simulink model "la_2dof_ctrl_obs"  (R2019b)
settings: Solver=FixedStepAuto  StartTime=0.0  StopTime=inf  FixedStep=0.001  RelTol=1e-3
model workspace (MAT data in the model file):
  SL_ROS_VariableLengthArrays_MaxSizes.CommonInfo.ArrayTruncateAction = 'EmitWarning'
  SL_ROS_VariableLengthArrays_MaxSizes.MsgTypeMap = containers.Map
  SL_ROS_VariableLengthArrays_MaxSizes.MsgTypeMap.serialization.keys = {'std_msgs/Float64MultiArray'}
  SL_ROS_VariableLengthArrays_MaxSizes.MsgTypeMap.serialization.values{1}.PropertyName = 'Data'
  SL_ROS_VariableLengthArrays_MaxSizes.MsgTypeMap.serialization.values{1}.DataType = 'double'
  SL_ROS_VariableLengthArrays_MaxSizes.MsgTypeMap.serialization.values{1}.MaxLength = 2
  SL_ROS_VariableLengthArrays_MaxSizes.MsgTypeMap.serialization.uniformity = 0
  SL_ROS_VariableLengthArrays_MaxSizes.MsgTypeMap.serialization.keyType = 'char'
  SL_ROS_VariableLengthArrays_MaxSizes.MsgTypeMap.serialization.valueType = 'any'
undefined symbols (not defined in the file): Data, Data_SL_Info
libraries: robotlib x6
settings Model: EnablePacing=on  Creator=markthemagnificent  LastModifiedBy=marco
settings OptimizationCC: EnhancedBackFolding=on  PassReuseOutputArgsAs=Individual arguments  ZeroExternalMemoryAtStartup=off  ZeroInternalMemoryAtStartup=off  MaxStackSize=64  OptimizeBlockOrder=speed  DifferentSizesBufferReuse=on  OptimizationCustomize=off  EfficientTunableParamExpr=on
settings DebuggingCC: ParameterTunabilityLossMsg=error
settings HardwareCC: ProdBitPerLong=64  ProdHWDeviceType=Intel->x86-64 (Linux 64)
settings SFSimCC: MATLABDynamicMemAlloc=off
settings RTWCC: SystemTargetFile=ert.tlc  HardwareBoard=Robot Operating System (ROS)  TLCOptions="-aInlineSetEventsForThisBaseRateFcn=TLC_FALSE -aSuppressMultiTaskScheduler=TLC_FALSE  -aRateBasedStepFcn=0"  TemplateMakefile=ert_default_tmf  GenerateReport=on  Toolchain=Catkin  IncludeHyperlinkInReport=on  LaunchReport=on  TargetLang=C++  GenerateTraceInfo=on  GenerateTraceReport=on  GenerateTraceReportSl=on  GenerateTraceReportSf=on  GenerateTraceReportEml=on
settings CodeAppCC: ForceParamTrailComments=on  IgnoreCustomStorageClasses=off  OperatorAnnotations=on  SimulinkDataObjDesc=on  SFDataObjDesc=on  InsertBlockDesc=on
settings ERTTargetCC: SupportContinuousTime=on

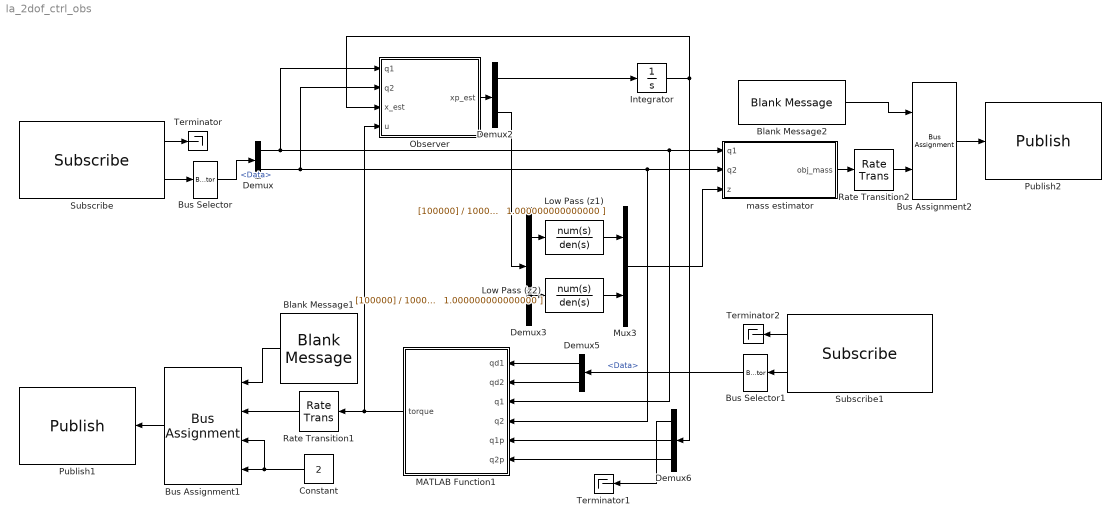
== system la_2dof_ctrl_obs ==
  Blank Message1 : robotlib/Blank Message  messageClass=Message  entityType=std_msgs/Float64MultiArray  messageType=std_msgs/Float64MultiArray  SampleTime=0.001
      settings: SourceProductName=ROS Toolbox
  Blank Message2 : robotlib/Blank Message  messageClass=Message  entityType=std_msgs/Float64  messageType=std_msgs/Float64  SampleTime=0.001
      settings: SourceProductName=ROS Toolbox
  Bus Assignment1 : BusAssignment  AssignedSignals=Data,Data_SL_Info.CurrentLength,Data_SL_Info.ReceivedLength
  Bus Assignment2 : BusAssignment  AssignedSignals=Data
  Bus Selector : BusSelector  OutputSignals=Data
  Bus Selector1 : BusSelector  OutputSignals=Data
  Constant : Constant  Value=2  OutDataTypeStr=uint32  SampleTime=0.001
  Demux : Demux  Outputs=2
  Demux2 : Demux  Outputs=[4,2]
  Demux3 : Demux  Outputs=2
  Demux5 : Demux  Outputs=2
  Demux6 : Demux  Outputs=[2,1,1]
  Integrator : Integrator  InitialCondition=[0 0 0 0]
  Low Pass (z1) : TransferFcn  Numerator=[100000]  Denominator=|
      | 100000*[0.000010000000000   0.000323606797750   0.005236067977500   0.052360679774998   0.323606797749979   1.000000000000000
      | ]
  Low Pass (z2) : TransferFcn  Numerator=[100000]  Denominator=|
      | 100000*[0.000010000000000   0.000323606797750   0.005236067977500   0.052360679774998   0.323606797749979   1.000000000000000
      | ]
  MATLAB Function1 : MATLAB Function  TreatAsAtomicUnit=on
  Mux3 : Mux  Inputs=2
  Observer : MATLAB Function  TreatAsAtomicUnit=on
  Publish1 : robotlib/Publish  topicSource=Specify your own  topic=/hardware/la_torque  messageType=std_msgs/Float64MultiArray  messageQueueLength=1
      settings: SourceProductName=ROS Toolbox
  Publish2 : robotlib/Publish  topicSource=Specify your own  topic=/hardware/la_estimated_mass  messageType=std_msgs/Float64  messageQueueLength=1
      settings: SourceProductName=ROS Toolbox
  Rate Transition1 : RateTransition
  Rate Transition2 : RateTransition
  Subscribe : robotlib/Subscribe  topicSource=Specify your own  topic=/hardware/la_current_pose  messageType=std_msgs/Float64MultiArray  sampleTime=0.001  messageQueueLength=1
      settings: SourceProductName=ROS Toolbox
  Subscribe1 : robotlib/Subscribe  topicSource=Specify your own  topic=/hardware/la_goal_pose  messageType=std_msgs/Float64MultiArray  sampleTime=0.001  messageQueueLength=1
      settings: SourceProductName=ROS Toolbox
  Terminator : Terminator
  Terminator1 : Terminator
  Terminator2 : Terminator
  mass estimator : MATLAB Function  TreatAsAtomicUnit=on
  wires:
  Integrator/1 -> Observer/3(x_est), Demux6/1
  Demux3/1 -> Low Pass (z1)/1
  Demux/2 -> MATLAB Function1/4(q2), mass estimator/2(q2), Observer/2(q2)
  Demux2/2 -> Demux3/1
  Demux2/1 -> Integrator/1
  Observer/1(xp_est) -> Demux2/1
  Demux3/2 -> Low Pass (z2)/1
  Low Pass (z1)/1 -> Mux3/1
  Low Pass (z2)/1 -> Mux3/2
  Mux3/1 -> mass estimator/3(z)
  MATLAB Function1/1(torque) -> Rate Transition1/1, Observer/4(u)
  Demux5/1 -> MATLAB Function1/1(qd1)
  Demux5/2 -> MATLAB Function1/2(qd2)
  Demux/1 -> MATLAB Function1/3(q1), mass estimator/1(q1), Observer/1(q1)
  Demux6/1 -> Terminator1/1
  Demux6/2 -> MATLAB Function1/5(q1p)
  Demux6/3 -> MATLAB Function1/6(q2p)
  Subscribe/1 -> Terminator/1
  Bus Selector/1 -> Demux/1  "<Data>"
  Subscribe/2 -> Bus Selector/1
  Subscribe1/1 -> Terminator2/1
  Subscribe1/2 -> Bus Selector1/1
  Bus Selector1/1 -> Demux5/1  "<Data>"
  Bus Assignment1/1 -> Publish1/1
  Rate Transition1/1 -> Bus Assignment1/2
  Constant/1 -> Bus Assignment1/3, Bus Assignment1/4
  Blank Message1/1 -> Bus Assignment1/1
  Bus Assignment2/1 -> Publish2/1
  mass estimator/1(obj_mass) -> Rate Transition2/1
  Rate Transition2/1 -> Bus Assignment2/2
  Blank Message2/1 -> Bus Assignment2/1

== matlab function la_2dof_ctrl_obs/mass estimator ==
  data: q1 input; q2 input; z input; obj_mass output
function obj_mass = mass_est(q1, q2, z)

obj_mass = 0;
%%% Physical parameters
length1  = 0.3303;
length2  = 0.4026;
lcenter1 = 0.165;
lcenter2 = 0.2113;
mass1    = 0.9;
mass2    = 1.2;
I1       = 0.9;
I2       = 1.2;
gravity  = 9.81;
%%%Some constants to reduce text space in matrix M
a1 = mass1*lcenter1^2 + mass2*length1^2 + mass2*lcenter2^2 + 2*mass2*length1*lcenter2^2 + I1 + I2;
a2 = 2*mass2*length1*lcenter2;
a3 = mass2*lcenter2^2 + I2;
a4 = mass2*length1*lcenter2;
a5 = mass2*lcenter2^2 + I2;
%%% Inertia matrix elements
m11 = a1 + a2*cos(q2);
m12 = a3 + a4*cos(q2);
m22 = a5;
%%%Matrices of the Lagrangian Model
M = [m11 m12; m12 m22];
phi = M * z;
if abs(sin(q1 + q2)) > 0.05
    obj_mass = -phi(2)/(length2*gravity*sin(q1 + q2));
else
    obj_mass = 0;
end

== matlab function la_2dof_ctrl_obs/MATLAB Function1 ==
  data: qd1 input; qd2 input; q1 input; q2 input; q1p input; q2p input; torque output
function torque = position_control(qd1,qd2,q1,q2,q1p,q2p)
length1  = 0.3303;
lcenter1 = 0.165;
lcenter2 = 0.1713;
mass1    = 0.9;
mass2    = 1.2;
gravity  = 9.81;

%%%Some constants to reduce text space in vector G
a7 = mass1*lcenter1*gravity + mass2*length1*gravity;
a8 = mass2*lcenter2*gravity;

g1 = a7*sin(qd1) + a8*sin(qd1 + qd2);
g2 = a8*sin(qd1 + qd2);
G = [g1; g2];

%%Constantes del control PD
kp=[7.5; 4.5];
kd=[3.5; 3.5];

qe= [qd1-q1; qd2-q2];

torque1 = G(1)+ kp(1)*qe(1)-kd(1)*q1p;
torque2 = G(2)+ kp(2)*qe(2)-kd(2)*q2p;

torque = [torque1; torque2];

== matlab function la_2dof_ctrl_obs/Observer ==
  data: q1 input; q2 input; x_est input; u input; xp_est output
function xp_est = observer(q1, q2, x_est, u)

xp_est = zeros(6,1);
q1_est  = x_est(1);
q2_est  = x_est(2);
q1p_est = x_est(3);
q2p_est = x_est(4);

%%NOMINAL DYNAMICS
%%% Physical parameters
length1  = 0.3303;
lcenter1 = 0.165;
lcenter2 = 0.2113;
mass1    = 0.9;
mass2    = 1.2;
I1       = 0.9;
I2       = 1.2;
gravity  = 9.81;
b1       = 1.5;
b2       = 1.5;
%%%Some constants to reduce text space in matrix M
a1 = mass1*lcenter1^2 + mass2*length1^2 + mass2*lcenter2^2 + 2*mass2*length1*lcenter2^2 + I1 + I2;
a2 = 2*mass2*length1*lcenter2;
a3 = mass2*lcenter2^2 + I2;
a4 = mass2*length1*lcenter2;
a5 = mass2*lcenter2^2 + I2;
%%%Some constants to reduce text space in matrix C
a6 = -mass2*length1*lcenter2;
%%%Some constants to reduce text space in vector G
a7 = mass1*lcenter1*gravity + mass2*length1*gravity;
a8 = mass2*lcenter2*gravity;
%%% Inertia matrix elements
m11 = a1 + a2*cos(q2);
m12 = a3 + a4*cos(q2);
m22 = a5;
%%% Coriolis matrix elements
c11 = a6*sin(q2)*q2p_est;
c12 = a6*sin(q2)*(q1p_est + q2p_est);
c21 = -a6*sin(q2)*q1p_est;
%%%Gravity elements
g1 = a7*sin(q1) + a8*sin(q1 + q2);
g2 = a8*sin(q1 + q2);
%%%Matrices of the Lagrangian Model
M = [m11 m12; m12 m22];
C = [c11 c12; c21 0];
G = [g1; g2];
B = [b1 0; 0 b2];
qpp_est = -M\((C + B)*[q1p_est; q2p_est] + G - u);
%%%

lambda = 5;
alpha  = 5;

z11 = lambda*sqrt(abs(q1 - q1_est))*sign(q1 - q1_est);
z12 = lambda*sqrt(abs(q2 - q2_est))*sign(q2 - q2_est);
z21 = alpha*sign(q1 - q1_est);
z22 = alpha*sign(q2 - q2_est);

xp_est(1) = q1p_est + z11;
xp_est(2) = q2p_est + z12;
xp_est(3) = qpp_est(1) + z21;
xp_est(4) = qpp_est(2) + z22;

xp_est(5) = z21;
xp_est(6) = z22;
